simulink model "forceEquation_withFeedback"  (R2024b)
settings: Solver=VariableStepAuto  StartTime=0.0  StopTime=10.0  RelTol=1e-3
values from neighbouring files (symbols this model uses):
  A = input("enter the value of A: ")    [forceEquation_withFeedback_mfile.m]
  F = input("enter the value of F: ")    [forceEquation_withFeedback_mfile.m]
  Ti = input("enter the value of Ti: ")    [forceEquation_withFeedback_mfile.m]
settings Model: Creator=admin  LastModifiedBy=admin

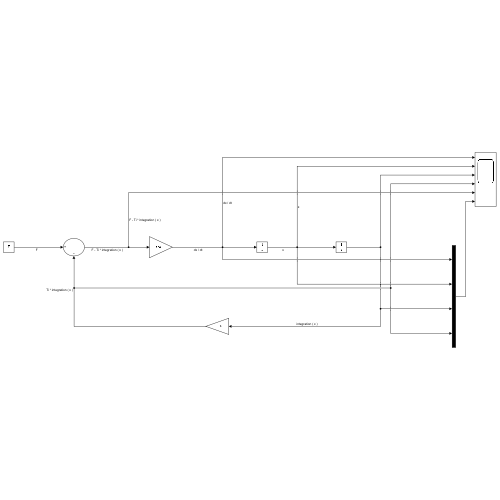
[thumbnail: Simulink's stored preview of the top-level diagram]
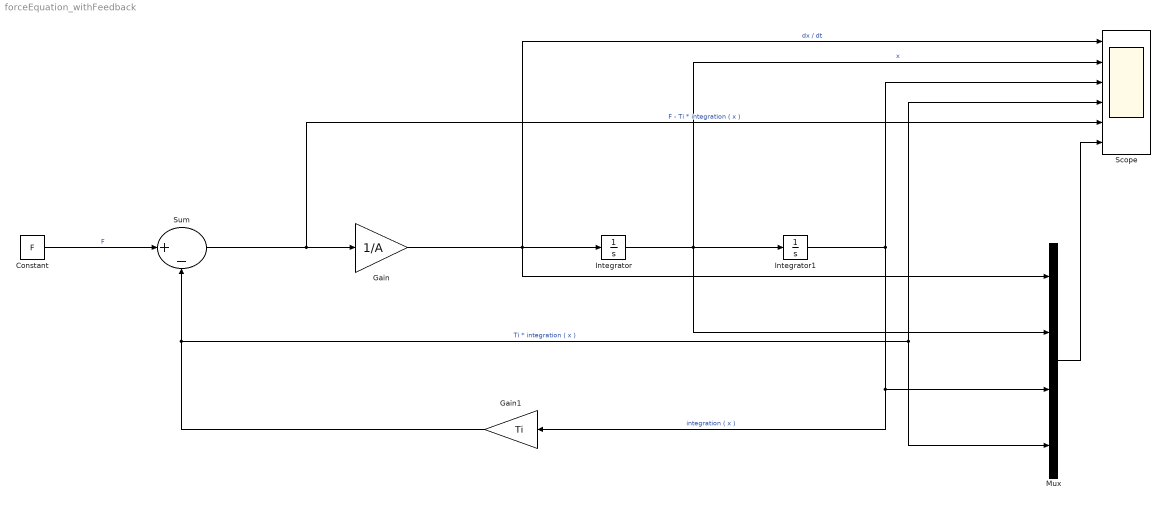
== system forceEquation_withFeedback ==
  Constant : Constant  Value=F
  Gain : Gain  Gain=1/A
  Gain1 : Gain  Gain=Ti
  Integrator : Integrator
  Integrator1 : Integrator
  Mux : Mux
  Scope : Scope  NumInputPorts=6
  Sum : Sum  Inputs=|+-
  wires:
  Integrator/1 -> Scope/2, Mux/2, Integrator1/1  "x"
  Gain/1 -> Mux/1, Scope/1, Integrator/1  "dx / dt"
  Integrator1/1 -> Gain1/1, Mux/3, Scope/3  "integration ( x )"
  Constant/1 -> Sum/1  "F"
  Gain1/1 -> Mux/4, Scope/4, Sum/2  "Ti * integration ( x )"
  Sum/1 -> Scope/5, Gain/1  "F - Ti * integration ( x )"
  Mux/1 -> Scope/6
